simulink model "qss_hybrid_electric_vehicle_DPM_FTP_75"  (R2022b)
settings: Solver=FixedStepAuto  StartTime=0.0  StopTime=1877  RelTol=1e-3  EnableMultiTasking=on
values from neighbouring files (symbols this model uses):
  time = 0:1:1877    [DP_FTP_75_main.m]    (also in output_visualization_FTP_75.m)
  u_in = u    [DP_FTP_75_main.m]    (also in output_visualization_FTP_75.m)
undefined symbols (not defined in the file or in its folder): H_u, rho_f
libraries: qss_tb_library x7
settings Model: Creator=d_goerges  LastModifiedBy=admin
settings SolverCC: AlgebraicLoopSolver=TrustRegion
settings DataIOCC: LimitDataPoints=on  SaveFormat=Array  SignalLoggingSaveFormat=ModelDataLogs  ReturnWorkspaceOutputs=off
settings OptimizationCC: ExpressionDepthLimit=2147483647  LifeSpan=inf
settings DebuggingCC: UnderspecifiedInitializationDetection=Classic  MergeDetectMultiDrivingBlocksExec=none  SolverPrmCheckMsg=warning  FcnCallInpInsideContextMsg=warning  UnconnectedInputMsg=warning  UnconnectedOutputMsg=warning  UnconnectedLineMsg=warning  StateNameClashWarn=warning  SFUnexpectedBacktrackingDiag=warning  SFNoUnconditionalDefaultTransitionDiag=warning  SFExecutionAtInitializationDiag=none  SFMachineParentedDataDiag=warning  ArithmeticOperatorsInVariantConditions=warning
settings HardwareCC: ProdBitPerPointer=32  ProdBitPerSizeT=32  ProdBitPerPtrDiffT=32  ProdLargestAtomicFloat=None  ProdIntDivRoundTo=Undefined  ProdEndianess=Unspecified  ProdWordSize=32  ProdHWDeviceType=32-bit Generic
settings ModelReferenceCC: EnableRefExpFcnMdlSchedulingChecks=on  PropagateSignalLabelsOutOfModel=off
settings SFSimCC: SimUseLocalCustomCode=off  CustomCodeUndefinedFunction=UseInterfaceOnly
settings RTWCC: RTWUseLocalCustomCode=off
settings CodeAppCC: StateflowObjectComments=on
settings GRTTargetCC: TargetLangStandard=C89/C90 (ANSI)  CombineOutputUpdateFcns=off  GRTInterface=on
settings ConfigComp: CovMetricSettings=dw  CovSaveCumulativeToWorkspaceVar=on  CovSaveSingleToWorkspaceVar=on  CovExternalEMLEnable=off

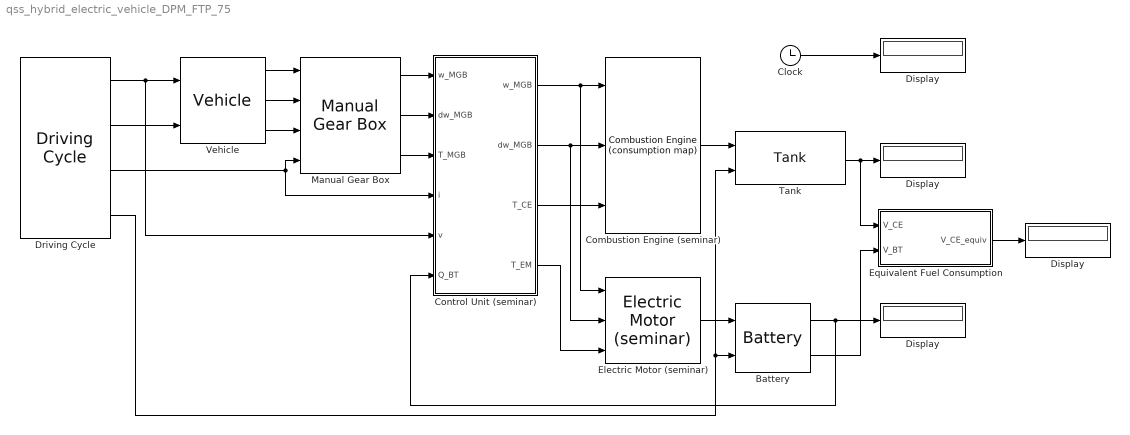
== system qss_hybrid_electric_vehicle_DPM_FTP_75 ==
  "   Display   " : Display
  "  Display  " : Display
  " Display " : Display
  Battery : qss_tb_library/Energy Buffer/Battery  Tag=battery  I_0=10  Q_BT_IC_rel=50  t_ch=2
  Clock : Clock
  Combustion Engine (seminar) : qss_tb_library/Energy Converter/Combustion Engine (consumption map)  Tag=combustion engine  theta_CE=0.2  w_CE_idle=105  P_CE_idle=8000  P_aux=0  ENABLE_FUEL_CUTOFF=on  T_CE_cutoff=5  P_CE_cutoff=0
  Control Unit (seminar) : Subsystem  Tag=control unit  mask(Control Unit){}
      mask help:
      | This block gives the user the opportunity to design his/her own control unit.
      |
      | The user can define the inputs and outputs  by himself/herself.
      mask init:
      | %init_control_unit;
  Display : Display
  Driving Cycle : qss_tb_library/Driving Cycle/Driving Cycle  Tag=cycle  cyclenr="USA:    FTP-75"  stepsize=1  autostop=on
  Electric Motor (seminar) : qss_tb_library/Energy Converter/Electric Motor (seminar)  theta_EM=0.1  P_aux=0
  Equivalent Fuel Consumption : Subsystem  mask(Equivalent Fuel Consumption){eta_BT=0.9, eta_EM=0.8, eta_CE=0.25}
      mask prompts: eta_BT "Battery efficiency [-]"; eta_EM "Motor efficiency [-]"; eta_CE "Engine efficiency [-]"
      mask help:
      | This block computes the equivalent fuel consumption.
      |
      | Input:
      | =====
      | 	V_CE    Fuel consumption [l/100 km]
      | 	V_BT    Energy consumption [kWh/100 km]
      |
      | Output:
      | ======
      | 	V_CE_equiv	Equivalent fuel consumption [l/100 km]
      mask init:
      | init_equivalent_fuel_consumption;
  Manual Gear Box : qss_tb_library/Gear System/Manual Gear Box  Tag=transmission  i_1=3.27  i_2=1.92  i_3=1.26  i_4=0.88  i_5=0.7  i_diff=3.29  e_GT=0.98  P_GT0=100  w_wheel_min=1
  Tank : qss_tb_library/Energy Source/Tank  Tag=tank  fuel=Diesel  flag_cold_start=on
  Vehicle : qss_tb_library/Vehicle/Vehicle  Tag=vehicle  m_f=1115  mt2m_f=5  A_f=2.3  d_wheel=0.576  cw=0.31  mu=0.013
  wires:
  Tank/1 -> Display/1, Equivalent Fuel Consumption/1(V_CE)
  Driving Cycle/2 -> Vehicle/2
  Driving Cycle/1 -> Vehicle/1, Control Unit (seminar)/5(v)
  Vehicle/1 -> Manual Gear Box/1
  Vehicle/2 -> Manual Gear Box/2
  Vehicle/3 -> Manual Gear Box/3
  Manual Gear Box/1 -> Control Unit (seminar)/1(w_MGB)
  Manual Gear Box/2 -> Control Unit (seminar)/2(dw_MGB)
  Manual Gear Box/3 -> Control Unit (seminar)/3(T_MGB)
  Control Unit (seminar)/1(" w_MGB ") -> Combustion Engine (seminar)/1, Electric Motor (seminar)/1
  Control Unit (seminar)/2(" dw_MGB ") -> Combustion Engine (seminar)/2, Electric Motor (seminar)/2
  Control Unit (seminar)/3(T_CE) -> Combustion Engine (seminar)/3
  Control Unit (seminar)/4(T_EM) -> Electric Motor (seminar)/3
  Combustion Engine (seminar)/1 -> Tank/1
  Electric Motor (seminar)/1 -> Battery/1
  Driving Cycle/4 -> Battery/2, Tank/2
  Battery/1 -> "  Display  "/1, Control Unit (seminar)/6(Q_BT)
  Driving Cycle/3 -> Manual Gear Box/4, Control Unit (seminar)/4(i)
  Battery/2 -> Equivalent Fuel Consumption/2(V_BT)
  Clock/1 -> " Display "/1
  Equivalent Fuel Consumption/1(V_CE_equiv) -> "   Display   "/1

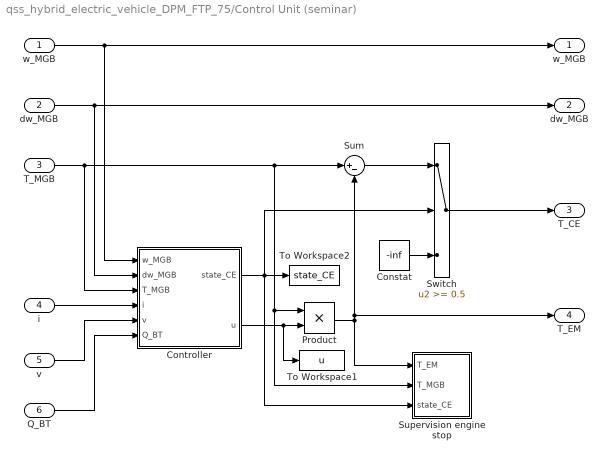
== system qss_hybrid_electric_vehicle_DPM_FTP_75/Control Unit (seminar) ==
  w_MGB : Inport
  dw_MGB : Inport  Port=2
  T_MGB : Inport  Port=3
  i : Inport  Port=4
  v : Inport  Port=5
  Q_BT : Inport  Port=6
  Constat : Constant  Value=-inf
  Controller : Subsystem  TreatAsAtomicUnit=on
  Product : Product  RndMeth=Zero
  Sum : Sum  Inputs=|+-
  Supervision engine stop : Subsystem
  Switch : Switch  Threshold=0.5  SaturateOnIntegerOverflow=off  InputSameDT=off
  To Workspace1 : ToWorkspace  VariableName=u  SampleTime=-1
  To Workspace2 : ToWorkspace  VariableName=state_CE  SampleTime=-1
  " w_MGB " : Outport  InitialOutput=0
  " dw_MGB " : Outport  Port=2  InitialOutput=0
  T_CE : Outport  Port=3  InitialOutput=0
  T_EM : Outport  Port=4  InitialOutput=0
  wires:
  dw_MGB/1 -> Controller/2(dw_MGB), " dw_MGB "/1
  w_MGB/1 -> Controller/1(w_MGB), " w_MGB "/1
  T_MGB/1 -> Controller/3(T_MGB), Sum/1, Product/1, Supervision engine stop/2(T_MGB)
  Product/1 -> Sum/2, T_EM/1, Supervision engine stop/1(T_EM)
  Controller/2(u) -> Product/2, To Workspace1/1
  i/1 -> Controller/4(i)
  Controller/1(state_CE) -> Switch/2, To Workspace2/1, Supervision engine stop/3(state_CE)
  Sum/1 -> Switch/1
  Switch/1 -> T_CE/1
  Constat/1 -> Switch/3
  v/1 -> Controller/5(v)
  Q_BT/1 -> Controller/6(Q_BT)

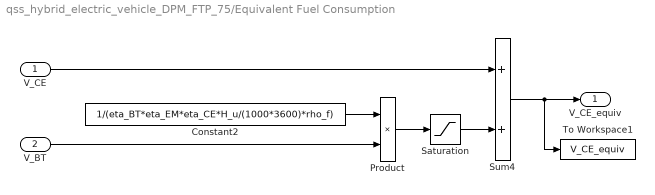
== system qss_hybrid_electric_vehicle_DPM_FTP_75/Equivalent Fuel Consumption ==
  V_CE : Inport
  V_BT : Inport  Port=2
  Constant2 : Constant  Value=1/(eta_BT*eta_EM*eta_CE*H_u/(1000*3600)*rho_f)
  Product : Product  RndMeth=Zero
  Saturation : Saturate  UpperLimit=inf  LowerLimit=0
  Sum4 : Sum  InputSameDT=on  SaturateOnIntegerOverflow=on  OutDataTypeStr=Inherit: Same as first input
  To Workspace1 : ToWorkspace  VariableName=V_CE_equiv  SampleTime=-1
  V_CE_equiv : Outport
  wires:
  Product/1 -> Saturation/1
  V_BT/1 -> Product/2
  Constant2/1 -> Product/1
  Sum4/1 -> To Workspace1/1, V_CE_equiv/1
  V_CE/1 -> Sum4/1
  Saturation/1 -> Sum4/2

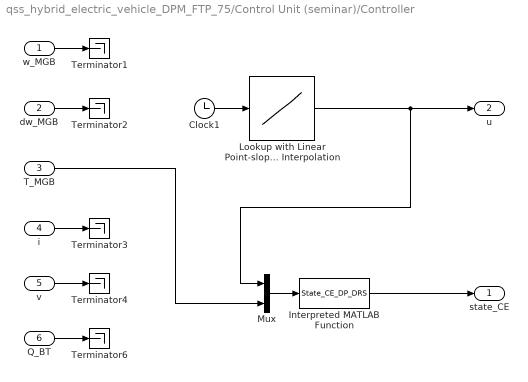
== system qss_hybrid_electric_vehicle_DPM_FTP_75/Control Unit (seminar)/Controller ==
  w_MGB : Inport
  dw_MGB : Inport  Port=2
  T_MGB : Inport  Port=3
  i : Inport  Port=4
  v : Inport  Port=5
  Q_BT : Inport  Port=6
  Clock1 : Clock
  Interpreted MATLAB Function : MATLABFcn  MATLABFcn=State_CE_DP_DRS
  Lookup with Linear Point-slope Interpolation : Lookup_n-D  NumberOfTableDimensions=1  BreakpointsForDimension1=time  Table=u_in  InternalRulePriority=Speed  RndMeth=Simplest
  Mux : Mux  Inputs=2
  Terminator{1..4,6} (5 alike) : Terminator
  state_CE : Outport  InitialOutput=0
  u : Outport  Port=2  InitialOutput=0
  wires:
  Q_BT/1 -> Terminator6/1
  dw_MGB/1 -> Terminator2/1
  i/1 -> Terminator3/1
  v/1 -> Terminator4/1
  w_MGB/1 -> Terminator1/1
  Clock1/1 -> Lookup with Linear Point-slope Interpolation/1
  Mux/1 -> Interpreted MATLAB Function/1
  Interpreted MATLAB Function/1 -> state_CE/1
  Lookup with Linear Point-slope Interpolation/1 -> Mux/1, u/1
  T_MGB/1 -> Mux/2

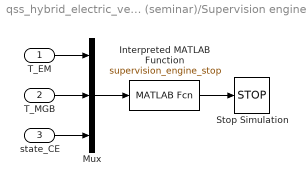
== system qss_hybrid_electric_vehicle_DPM_FTP_75/Control Unit (seminar)/Supervision engine stop ==
  T_EM : Inport
  T_MGB : Inport  Port=2
  state_CE : Inport  Port=3
  Interpreted MATLAB Function : MATLABFcn  MATLABFcn=supervision_engine_stop
  Mux : Mux  Inputs=3
  Stop Simulation : Stop
  wires:
  T_MGB/1 -> Mux/2
  T_EM/1 -> Mux/1
  state_CE/1 -> Mux/3
  Mux/1 -> Interpreted MATLAB Function/1
  Interpreted MATLAB Function/1 -> Stop Simulation/1
